simulink model "exclusive_or"  (R2022a)
settings: Solver=VariableStepAuto  StartTime=0.0  StopTime=10.0  RelTol=1e-3
settings Model: Creator=q541028  LastModifiedBy=q541028

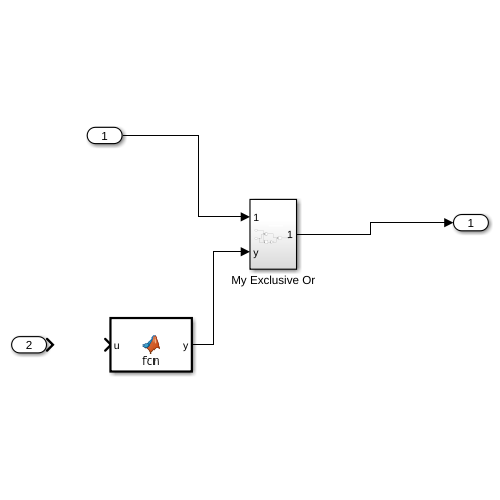
[thumbnail: Simulink's stored preview of the top-level diagram]
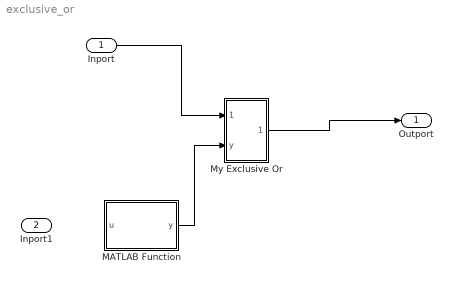
== system exclusive_or ==
  Inport : Inport
  Inport1 : Inport  Port=2
  MATLAB Function : MATLAB Function  TreatAsAtomicUnit=on
  My Exclusive Or : Subsystem
  Outport : Outport
  wires:
  Inport/1 -> My Exclusive Or/1(In1)
  My Exclusive Or/1(Out1) -> Outport/1
  MATLAB Function/1(y) -> My Exclusive Or/2(y)

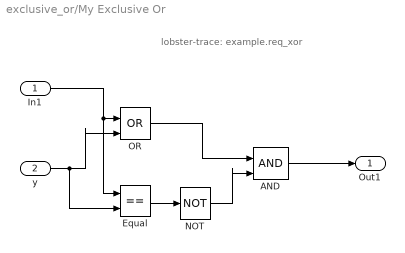
== system exclusive_or/My Exclusive Or ==
  note: lobster-trace: example.req_xor
  In1 : Inport
  y : Inport  Port=2
  AND : Logic  IconShape=distinctive  AllPortsSameDT=off  OutDataTypeStr=boolean
  Equal : RelationalOperator  Operator===  OutDataTypeStr=boolean  RndMeth=Simplest  InputSameDT=off
  NOT : Logic  Operator=NOT  IconShape=distinctive  AllPortsSameDT=off  OutDataTypeStr=boolean
  OR : Logic  Operator=OR  IconShape=distinctive  AllPortsSameDT=off  OutDataTypeStr=boolean
  Out1 : Outport
  wires:
  Equal/1 -> NOT/1
  AND/1 -> Out1/1
  NOT/1 -> AND/2
  OR/1 -> AND/1
  In1/1 -> Equal/1, OR/1
  y/1 -> Equal/2, OR/2

== matlab function exclusive_or/MATLAB Function ==
  data: u input; y output
function y = fcn(u)

y = u;
